simulink subsystem "rss_HWOvrCurrDia"  (R2023a)
settings: Solver=VariableStepAuto  StartTime=0.0  StopTime=10.0  RelTol=1e-3
undefined symbols (not defined in the file): ENM_TYPE_FALT, Gu16_ctHWOvrCurrConfCnt_C, Gu16_ctHWOvrCurrRcvyCnt_C
libraries: lib_debounce x1, lib_fault_definiteness x1
settings Model: Creator=xiaoqiang.yuan  LastModifiedBy=xiaoqiang.yuan

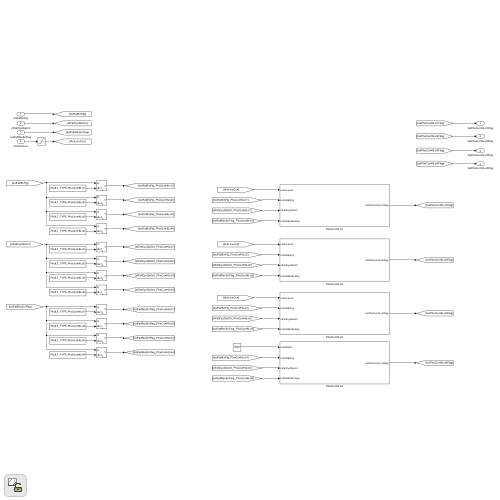
[thumbnail: Simulink's stored preview of the top-level diagram]
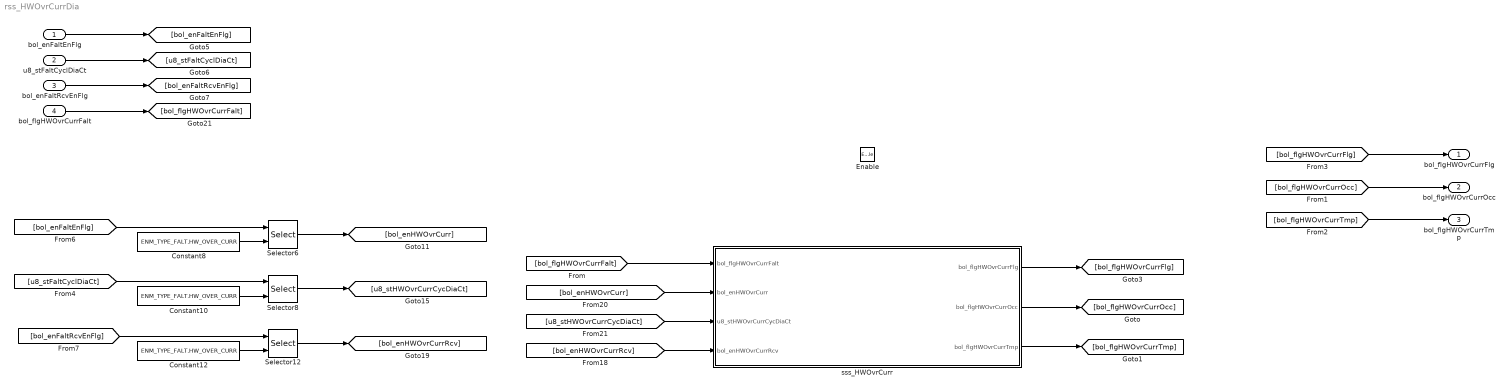
== system rss_HWOvrCurrDia ==
  bol_enFaltEnFlg : Inport  OutDataTypeStr=boolean
  u8_stFaltCyclDiaCt : Inport  Port=2  OutDataTypeStr=uint8
  bol_enFaltRcvEnFlg : Inport  Port=3  OutDataTypeStr=boolean
  bol_flgHWOvrCurrFalt : Inport  Port=4  OutDataTypeStr=boolean
  Enable : EnablePort
  Constant10 : Constant  Value=ENM_TYPE_FALT.HW_OVER_CURR
  Constant12 : Constant  Value=ENM_TYPE_FALT.HW_OVER_CURR
  Constant8 : Constant  Value=ENM_TYPE_FALT.HW_OVER_CURR
  Selector12 : Selector  IndexMode=Zero-based  InputPortWidth=Cdbl_numFaltDiaNum  IndexOptions=Index vector (port)  Indices=[1 3]  OutputSizes=1
  Selector6 : Selector  IndexMode=Zero-based  InputPortWidth=Cdbl_numFaltDiaNum  IndexOptions=Index vector (port)  Indices=[1 3]  OutputSizes=1
  Selector8 : Selector  IndexMode=Zero-based  InputPortWidth=Cdbl_numFaltDiaNum  IndexOptions=Index vector (port)  Indices=[1 3]  OutputSizes=1
  sss_HWOvrCurr : Subsystem
  bol_flgHWOvrCurrFlg : Outport  OutDataTypeStr=boolean
  bol_flgHWOvrCurrOcc : Outport  Port=2  OutDataTypeStr=boolean  InitialOutput=0
  bol_flgHWOvrCurrTmp : Outport  Port=3  OutDataTypeStr=boolean  InitialOutput=0
  wires:
  [bol_flgHWOvrCurrFlg] -> bol_flgHWOvrCurrFlg/1
  bol_enFaltEnFlg/1 -> [bol_enFaltEnFlg]
  [u8_stFaltCyclDiaCt] -> Selector8/1
  u8_stFaltCyclDiaCt/1 -> [u8_stFaltCyclDiaCt]
  bol_enFaltRcvEnFlg/1 -> [bol_enFaltRcvEnFlg]
  [bol_enFaltEnFlg] -> Selector6/1
  Constant8/1 -> Selector6/2
  Constant10/1 -> Selector8/2
  [bol_enFaltRcvEnFlg] -> Selector12/1
  Constant12/1 -> Selector12/2
  Selector6/1 -> [bol_enHWOvrCurr]
  Selector8/1 -> [u8_stHWOvrCurrCycDiaCt]
  Selector12/1 -> [bol_enHWOvrCurrRcv]
  sss_HWOvrCurr/1(bol_flgHWOvrCurrFlg) -> [bol_flgHWOvrCurrFlg]
  [bol_enHWOvrCurrRcv] -> sss_HWOvrCurr/4(bol_enHWOvrCurrRcv)
  [u8_stHWOvrCurrCycDiaCt] -> sss_HWOvrCurr/3(u8_stHWOvrCurrCycDiaCt)
  [bol_enHWOvrCurr] -> sss_HWOvrCurr/2(bol_enHWOvrCurr)
  [bol_flgHWOvrCurrFalt] -> sss_HWOvrCurr/1(bol_flgHWOvrCurrFalt)
  bol_flgHWOvrCurrFalt/1 -> [bol_flgHWOvrCurrFalt]
  [bol_flgHWOvrCurrOcc] -> bol_flgHWOvrCurrOcc/1
  sss_HWOvrCurr/2(bol_flgHWOvrCurrOcc) -> [bol_flgHWOvrCurrOcc]
  [bol_flgHWOvrCurrTmp] -> bol_flgHWOvrCurrTmp/1
  sss_HWOvrCurr/3(bol_flgHWOvrCurrTmp) -> [bol_flgHWOvrCurrTmp]

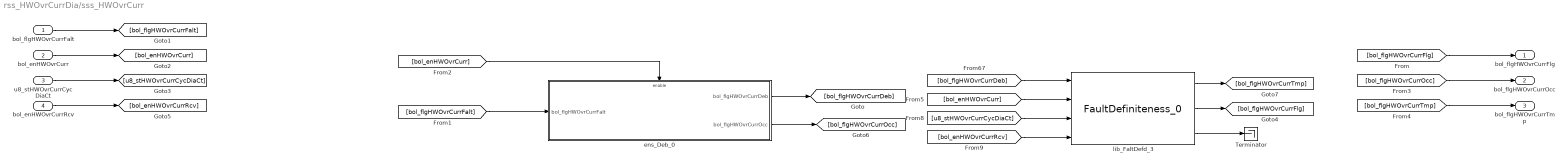
== system rss_HWOvrCurrDia/sss_HWOvrCurr ==
  bol_flgHWOvrCurrFalt : Inport
  bol_enHWOvrCurr : Inport  Port=2
  u8_stHWOvrCurrCycDiaCt : Inport  Port=3
  bol_enHWOvrCurrRcv : Inport  Port=4
  Terminator : Terminator
  ens_Deb_0 : Subsystem
  lib_FaltDefd_3 : lib_fault_definiteness/FaultDefiniteness_0  lb_FaltWaitRecvCnt=Gu16_ctHWOvrCurrConfCnt_C
  bol_flgHWOvrCurrFlg : Outport
  bol_flgHWOvrCurrOcc : Outport  Port=2  OutputWhenDisabled=reset  InitialOutput=0
  bol_flgHWOvrCurrTmp : Outport  Port=3  InitialOutput=0
  wires:
  [bol_flgHWOvrCurrTmp] -> bol_flgHWOvrCurrTmp/1
  ens_Deb_0/2(bol_flgHWOvrCurrOcc) -> [bol_flgHWOvrCurrOcc]
  [bol_flgHWOvrCurrOcc] -> bol_flgHWOvrCurrOcc/1
  bol_flgHWOvrCurrFalt/1 -> [bol_flgHWOvrCurrFalt]
  [bol_flgHWOvrCurrFalt] -> ens_Deb_0/1(bol_flgHWOvrCurrFalt)
  lib_FaltDefd_3/1 -> [bol_flgHWOvrCurrTmp]
  lib_FaltDefd_3/2 -> [bol_flgHWOvrCurrFlg]
  lib_FaltDefd_3/3 -> Terminator/1
  [bol_flgHWOvrCurrDeb] -> lib_FaltDefd_3/1
  [bol_enHWOvrCurr] -> lib_FaltDefd_3/2
  [u8_stHWOvrCurrCycDiaCt] -> lib_FaltDefd_3/3
  [bol_enHWOvrCurrRcv] -> lib_FaltDefd_3/4
  [bol_flgHWOvrCurrFlg] -> bol_flgHWOvrCurrFlg/1
  bol_enHWOvrCurr/1 -> [bol_enHWOvrCurr]
  u8_stHWOvrCurrCycDiaCt/1 -> [u8_stHWOvrCurrCycDiaCt]
  bol_enHWOvrCurrRcv/1 -> [bol_enHWOvrCurrRcv]
  ens_Deb_0/1(bol_flgHWOvrCurrDeb) -> [bol_flgHWOvrCurrDeb]
  [bol_enHWOvrCurr] -> ens_Deb_0/Enable

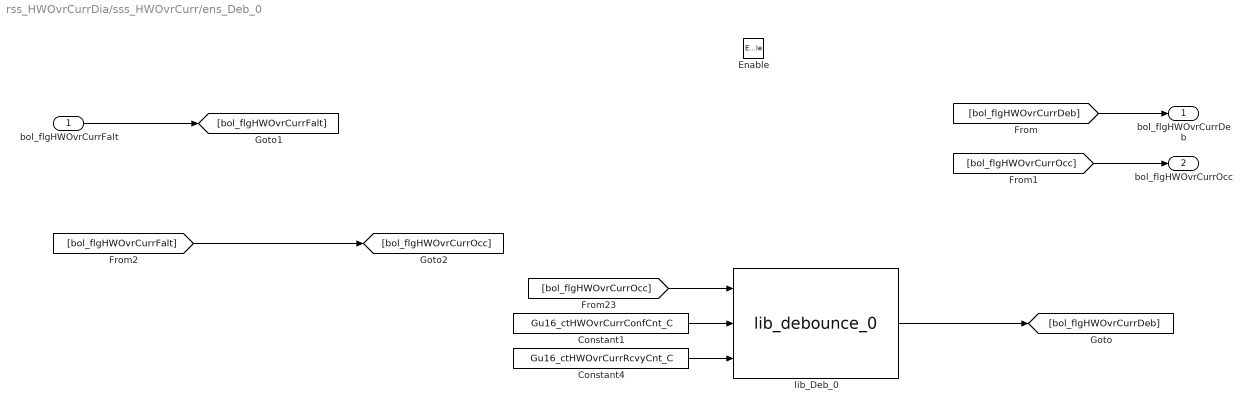
== system rss_HWOvrCurrDia/sss_HWOvrCurr/ens_Deb_0 ==
  bol_flgHWOvrCurrFalt : Inport
  Enable : EnablePort
  Constant1 : Constant  Value=Gu16_ctHWOvrCurrConfCnt_C
  Constant4 : Constant  Value=Gu16_ctHWOvrCurrRcvyCnt_C
  lib_Deb_0 : lib_debounce/lib_debounce_0
  bol_flgHWOvrCurrDeb : Outport
  bol_flgHWOvrCurrOcc : Outport  Port=2
  wires:
  [bol_flgHWOvrCurrFalt] -> [bol_flgHWOvrCurrOcc]
  [bol_flgHWOvrCurrOcc] -> bol_flgHWOvrCurrOcc/1
  [bol_flgHWOvrCurrOcc] -> lib_Deb_0/1
  lib_Deb_0/1 -> [bol_flgHWOvrCurrDeb]
  bol_flgHWOvrCurrFalt/1 -> [bol_flgHWOvrCurrFalt]
  [bol_flgHWOvrCurrDeb] -> bol_flgHWOvrCurrDeb/1
  Constant4/1 -> lib_Deb_0/3
  Constant1/1 -> lib_Deb_0/2
